simulink model "Motor_position_control"  (R2020b)
settings: Solver=VariableStepAuto  StartTime=0.0  StopTime=10.0  RelTol=1e-3
values from neighbouring files (symbols this model uses):
  J = 3.228E-6    (= 3.228e-06)    [variable.m]
  L = 2.74e-4    (= 0.000274)    [variable.m]
  R = 4    [variable.m]
undefined symbols (not defined in the file or in its folder): B, Kb, Kt
settings Model: Creator=sonal  LastModifiedBy=sonal

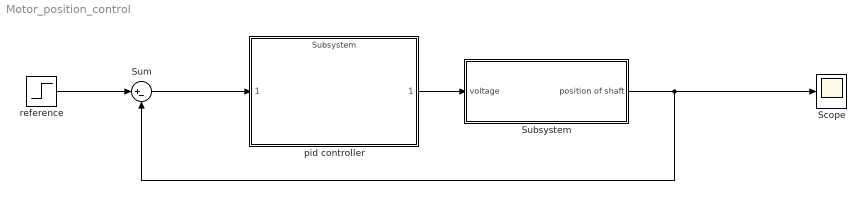
== system Motor_position_control ==
  Scope : Scope
  Subsystem : Subsystem
  Sum : Sum  Inputs=|+-
  pid controller : ModelReference  ModelNameDialog=Subsystem  SimulationMode=Normal  ModelReferenceVersion=1.3
  "reference " : Step  Time=0  SampleTime=0
  wires:
  Subsystem/1(position of shaft) -> Scope/1, Sum/2
  Sum/1 -> pid controller/1
  pid controller/1 -> Subsystem/1(voltage)
  "reference "/1 -> Sum/1

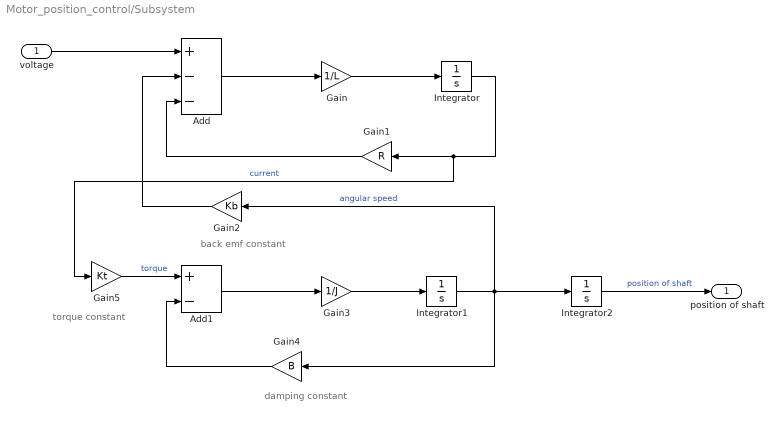
== system Motor_position_control/Subsystem ==
  note: torque constant
  note: back emf constant
  note: damping constant
  voltage : Inport
  Add : Sum  Inputs=+--
  Add1 : Sum  Inputs=+-
  Gain : Gain  Gain=1/L
  Gain1 : Gain  Gain=R
  Gain2 : Gain  Gain=Kb
  Gain3 : Gain  Gain=1/J
  Gain4 : Gain  Gain=B
  Gain5 : Gain  Gain=Kt
  Integrator : Integrator
  Integrator1 : Integrator
  Integrator2 : Integrator
  position of shaft : Outport
  wires:
  Add/1 -> Gain/1
  Gain1/1 -> Add/3
  Gain/1 -> Integrator/1
  Gain3/1 -> Integrator1/1
  Gain2/1 -> Add/2
  Integrator/1 -> Gain5/1, Gain1/1  "current"
  Add1/1 -> Gain3/1
  Gain4/1 -> Add1/2
  Gain5/1 -> Add1/1  "torque"
  Integrator1/1 -> Gain4/1, Gain2/1, Integrator2/1  "angular speed"
  voltage/1 -> Add/1
  Integrator2/1 -> position of shaft/1  "position of shaft"
